simulink model "SecRwLtStLgrstUpwdDnwdCtrl"  (R2018b)
settings: Solver=FixedStepDiscrete  StartTime=0.0  StopTime=10.0  FixedStep=0.01  RelTol=1e-3
undefined symbols (not defined in the file or in its folder): KeSMSuMdMotFinshdTm_Val, KeSMSuMdRetryTm1_Val, KeSMSuModeReqDurgTm_Val, KeSMSwSecRwLtStLgrstUpwdDnwdEnTrigBitMask_Val
libraries: StCtrlLibBkRecln x1
settings Model: Creator=sn2xws  LastModifiedBy=sn55gm
settings Model: ModifiedHistory=|
  | 2024.10.14 V3.0.0 bitmask接口改为变量接口
  | 25.7.7 V3.13.0 Md61 Md62新增Retry口
settings DataIOCC: SaveFormat=StructureWithTime
settings OptimizationCC: DefaultParameterBehavior=Inlined  EnhancedBackFolding=on  PassReuseOutputArgsAs=Individual arguments  ZeroExternalMemoryAtStartup=off  ZeroInternalMemoryAtStartup=off  OptimizeBlockOrder=speed  DifferentSizesBufferReuse=on  OptimizationCustomize=off
settings DebuggingCC: ParameterTunabilityLossMsg=error
settings ModelReferenceCC: ModelReferenceNumInstancesAllowed=Single
settings SFSimCC: MATLABDynamicMemAlloc=off
settings RTWCC: SystemTargetFile=autosar.tlc  GenCodeOnly=on  TemplateMakefile=ert_default_tmf  Description=AUTOSAR  GenerateReport=on  IncludeHyperlinkInReport=on  LaunchReport=on  GenerateTraceInfo=on  GenerateTraceReport=on  GenerateTraceReportSl=on  GenerateTraceReportSf=on  GenerateTraceReportEml=on
settings CodeAppCC: ForceParamTrailComments=on  IgnoreCustomStorageClasses=off  OperatorAnnotations=on  SimulinkDataObjDesc=on  SFDataObjDesc=on  InsertBlockDesc=on
settings STFCustomTargetCC: TargetLangStandard=C99 (ISO)  MultiwordLength=256  ParMdlRefBuildCompliant=on  CompOptLevelCompliant=on  IncludeMdlTerminateFcn=off  CombineOutputUpdateFcns=on  SuppressErrorStatus=on  ERTCustomFileBanners=on  SupportNonFinite=off  SupportComplex=off  SupportContinuousTime=off  SupportNonInlinedSFcns=off  RemoveResetFunc=on  MATLABClassNameForMDSCustomization=Simulink.SoftwareTarget.ERTCustomization  AutosarCompliant=on  UseToolchainInfoCompliant=on  LookupTableObjectStructAxisOrder=2,1,3,4,...  LUTObjectStructOrderEvenSpacing=Size,Table,Breakpoints  SystemTargetFile=autosar.tlc
settings ERTTargetCC: TargetLangStandard=C99 (ISO)  ConcurrentExecutionCompliant=off  IncludeMdlTerminateFcn=off  SuppressErrorStatus=on  SupportNonFinite=off  SupportComplex=off  ModelStepFunctionPrototypeControlCompliant=off  CPPClassGenCompliant=off  AutosarCompliant=on  LookupTableObjectStructAxisOrder=2,1,3,4,...  LUTObjectStructOrderEvenSpacing=Size,Table,Breakpoints  InlinedParameterPlacement=NonHierarchical  ERTCustomFileTemplate=example_file_process.tlc  ERTFilePackagingFormat=Compact

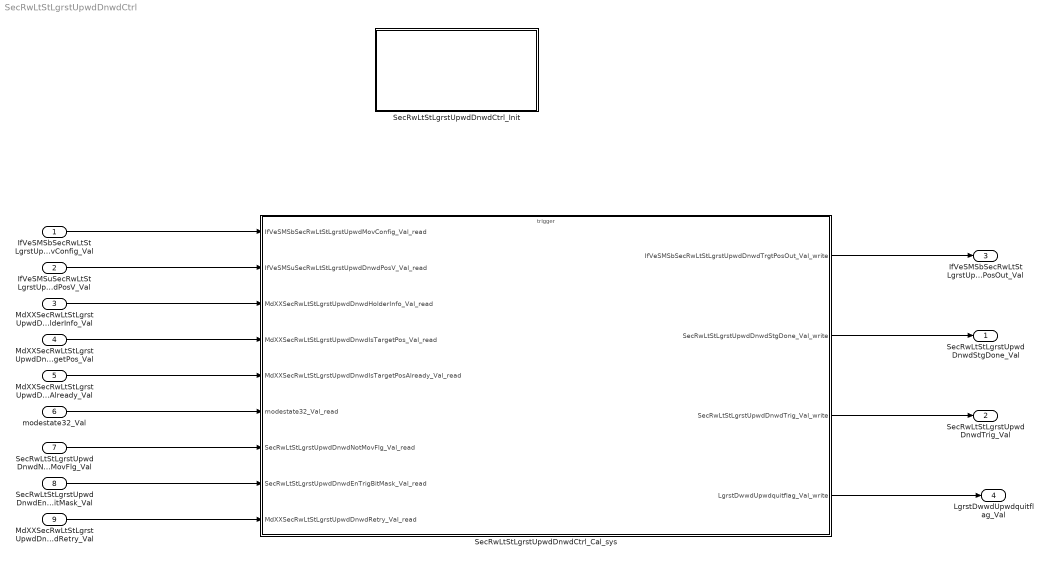
== system SecRwLtStLgrstUpwdDnwdCtrl ==
  IfVeSMSbSecRwLtStLgrstUpwdMovConfig_Val : Inport  OutDataTypeStr=boolean  PortDimensions=1
  IfVeSMSuSecRwLtStLgrstUpwdDnwdPosV_Val : Inport  Port=2  OutDataTypeStr=boolean  PortDimensions=1
  MdXXSecRwLtStLgrstUpwdDnwdHolderInfo_Val : Inport  Port=3  OutDataTypeStr=uint32  PortDimensions=1
  MdXXSecRwLtStLgrstUpwdDnwdIsTargetPos_Val : Inport  Port=4  OutDataTypeStr=uint32  PortDimensions=1
  MdXXSecRwLtStLgrstUpwdDnwdIsTargetPosAlready_Val : Inport  Port=5  OutDataTypeStr=uint32  PortDimensions=1
  modestate32_Val : Inport  Port=6  OutDataTypeStr=uint32  PortDimensions=1
  SecRwLtStLgrstUpwdDnwdNotMovFlg_Val : Inport  Port=7  OutDataTypeStr=boolean  PortDimensions=1
  SecRwLtStLgrstUpwdDnwdEnTrigBitMask_Val : Inport  Port=8  OutDataTypeStr=uint32  PortDimensions=1
  MdXXSecRwLtStLgrstUpwdDnwdRetry_Val : Inport  Port=9  OutDataTypeStr=uint32  PortDimensions=1
  SecRwLtStLgrstUpwdDnwdCtrl_Cal_sys : Subsystem
  SecRwLtStLgrstUpwdDnwdCtrl_Init : Subsystem
  SecRwLtStLgrstUpwdDnwdStgDone_Val : Outport  OutDataTypeStr=boolean  PortDimensions=1
  SecRwLtStLgrstUpwdDnwdTrig_Val : Outport  Port=2  OutDataTypeStr=boolean  PortDimensions=1
  IfVeSMSbSecRwLtStLgrstUpwdDnwdTrgtPosOut_Val : Outport  Port=3  OutDataTypeStr=boolean  PortDimensions=1
  LgrstDwwdUpwdquitflag_Val : Outport  Port=4  OutDataTypeStr=boolean  PortDimensions=1
  wires:
  IfVeSMSbSecRwLtStLgrstUpwdMovConfig_Val/1 -> SecRwLtStLgrstUpwdDnwdCtrl_Cal_sys/1(IfVeSMSbSecRwLtStLgrstUpwdMovConfig_Val_read)
  IfVeSMSuSecRwLtStLgrstUpwdDnwdPosV_Val/1 -> SecRwLtStLgrstUpwdDnwdCtrl_Cal_sys/2(IfVeSMSuSecRwLtStLgrstUpwdDnwdPosV_Val_read)
  MdXXSecRwLtStLgrstUpwdDnwdHolderInfo_Val/1 -> SecRwLtStLgrstUpwdDnwdCtrl_Cal_sys/3(MdXXSecRwLtStLgrstUpwdDnwdHolderInfo_Val_read)
  MdXXSecRwLtStLgrstUpwdDnwdIsTargetPos_Val/1 -> SecRwLtStLgrstUpwdDnwdCtrl_Cal_sys/4(MdXXSecRwLtStLgrstUpwdDnwdIsTargetPos_Val_read)
  MdXXSecRwLtStLgrstUpwdDnwdIsTargetPosAlready_Val/1 -> SecRwLtStLgrstUpwdDnwdCtrl_Cal_sys/5(MdXXSecRwLtStLgrstUpwdDnwdIsTargetPosAlready_Val_read)
  modestate32_Val/1 -> SecRwLtStLgrstUpwdDnwdCtrl_Cal_sys/6(modestate32_Val_read)
  SecRwLtStLgrstUpwdDnwdNotMovFlg_Val/1 -> SecRwLtStLgrstUpwdDnwdCtrl_Cal_sys/7(SecRwLtStLgrstUpwdDnwdNotMovFlg_Val_read)
  SecRwLtStLgrstUpwdDnwdCtrl_Cal_sys/1(IfVeSMSbSecRwLtStLgrstUpwdDnwdTrgtPosOut_Val_write) -> IfVeSMSbSecRwLtStLgrstUpwdDnwdTrgtPosOut_Val/1
  SecRwLtStLgrstUpwdDnwdCtrl_Cal_sys/2(SecRwLtStLgrstUpwdDnwdStgDone_Val_write) -> SecRwLtStLgrstUpwdDnwdStgDone_Val/1
  SecRwLtStLgrstUpwdDnwdCtrl_Cal_sys/3(SecRwLtStLgrstUpwdDnwdTrig_Val_write) -> SecRwLtStLgrstUpwdDnwdTrig_Val/1
  SecRwLtStLgrstUpwdDnwdEnTrigBitMask_Val/1 -> SecRwLtStLgrstUpwdDnwdCtrl_Cal_sys/8(SecRwLtStLgrstUpwdDnwdEnTrigBitMask_Val_read)
  MdXXSecRwLtStLgrstUpwdDnwdRetry_Val/1 -> SecRwLtStLgrstUpwdDnwdCtrl_Cal_sys/9(MdXXSecRwLtStLgrstUpwdDnwdRetry_Val_read)
  SecRwLtStLgrstUpwdDnwdCtrl_Cal_sys/4(LgrstDwwdUpwdquitflag_Val_write) -> LgrstDwwdUpwdquitflag_Val/1

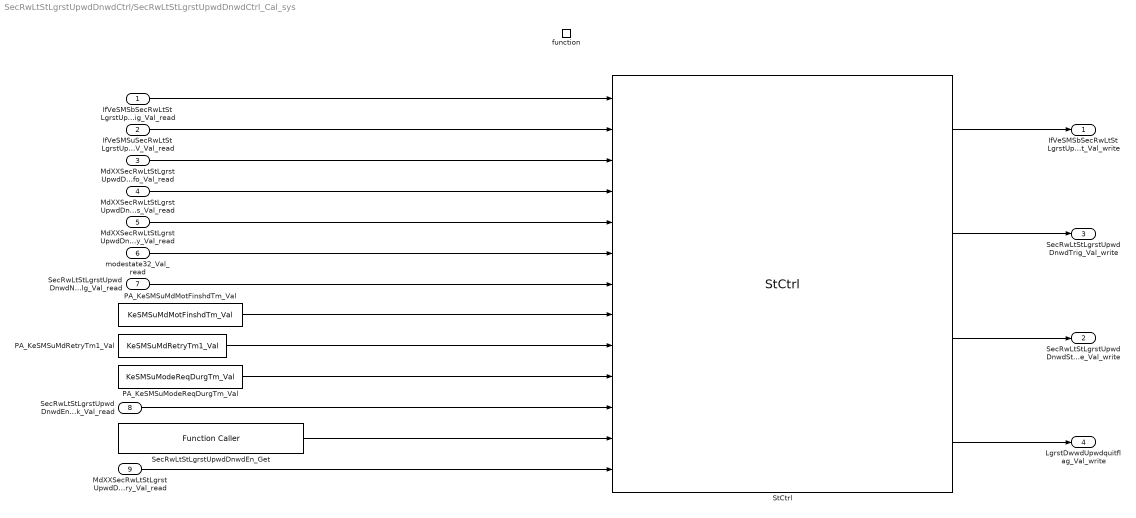
== system SecRwLtStLgrstUpwdDnwdCtrl/SecRwLtStLgrstUpwdDnwdCtrl_Cal_sys ==
  IfVeSMSbSecRwLtStLgrstUpwdMovConfig_Val_read : Inport
  IfVeSMSuSecRwLtStLgrstUpwdDnwdPosV_Val_read : Inport  Port=2
  MdXXSecRwLtStLgrstUpwdDnwdHolderInfo_Val_read : Inport  Port=3
  MdXXSecRwLtStLgrstUpwdDnwdIsTargetPos_Val_read : Inport  Port=4
  MdXXSecRwLtStLgrstUpwdDnwdIsTargetPosAlready_Val_read : Inport  Port=5
  modestate32_Val_read : Inport  Port=6
  SecRwLtStLgrstUpwdDnwdNotMovFlg_Val_read : Inport  Port=7
  SecRwLtStLgrstUpwdDnwdEnTrigBitMask_Val_read : Inport  Port=8
  MdXXSecRwLtStLgrstUpwdDnwdRetry_Val_read : Inport  Port=9
  function : TriggerPort  TriggerType=function-call  IsSimulinkFunction=on  FunctionName=SecRwLtStLgrstUpwdDnwdCtrl_Cal  VariantControl=(inherit)
  PA_KeSMSuMdMotFinshdTm_Val : Constant  Value=KeSMSuMdMotFinshdTm_Val
  PA_KeSMSuMdRetryTm1_Val : Constant  Value=KeSMSuMdRetryTm1_Val
  PA_KeSMSuModeReqDurgTm_Val : Constant  Value=KeSMSuModeReqDurgTm_Val
  SecRwLtStLgrstUpwdDnwdEn_Get : FunctionCaller  FunctionPrototype=data = SecRwLtStLgrstUpwdDnwdEn_Get()  OutputArgumentSpecifications=uint32(1)
  StCtrl : StCtrlLibBkRecln/StCtrl  SystemSampleTime=-1
  IfVeSMSbSecRwLtStLgrstUpwdDnwdTrgtPosOut_Val_write : Outport
      settings: EnsureOutportIsVirtual=on
  SecRwLtStLgrstUpwdDnwdStgDone_Val_write : Outport  Port=2
      settings: EnsureOutportIsVirtual=on
  SecRwLtStLgrstUpwdDnwdTrig_Val_write : Outport  Port=3
      settings: EnsureOutportIsVirtual=on
  LgrstDwwdUpwdquitflag_Val_write : Outport  Port=4
      settings: EnsureOutportIsVirtual=on
  wires:
  StCtrl/1 -> IfVeSMSbSecRwLtStLgrstUpwdDnwdTrgtPosOut_Val_write/1
  StCtrl/2 -> SecRwLtStLgrstUpwdDnwdTrig_Val_write/1
  StCtrl/3 -> SecRwLtStLgrstUpwdDnwdStgDone_Val_write/1
  IfVeSMSbSecRwLtStLgrstUpwdMovConfig_Val_read/1 -> StCtrl/1
  IfVeSMSuSecRwLtStLgrstUpwdDnwdPosV_Val_read/1 -> StCtrl/2
  MdXXSecRwLtStLgrstUpwdDnwdHolderInfo_Val_read/1 -> StCtrl/3
  MdXXSecRwLtStLgrstUpwdDnwdIsTargetPos_Val_read/1 -> StCtrl/4
  MdXXSecRwLtStLgrstUpwdDnwdIsTargetPosAlready_Val_read/1 -> StCtrl/5
  modestate32_Val_read/1 -> StCtrl/6
  SecRwLtStLgrstUpwdDnwdNotMovFlg_Val_read/1 -> StCtrl/7
  SecRwLtStLgrstUpwdDnwdEnTrigBitMask_Val_read/1 -> StCtrl/11
  SecRwLtStLgrstUpwdDnwdEn_Get/1 -> StCtrl/12
  PA_KeSMSuMdMotFinshdTm_Val/1 -> StCtrl/8
  PA_KeSMSuModeReqDurgTm_Val/1 -> StCtrl/10
  PA_KeSMSuMdRetryTm1_Val/1 -> StCtrl/9
  MdXXSecRwLtStLgrstUpwdDnwdRetry_Val_read/1 -> StCtrl/13
  StCtrl/4 -> LgrstDwwdUpwdquitflag_Val_write/1

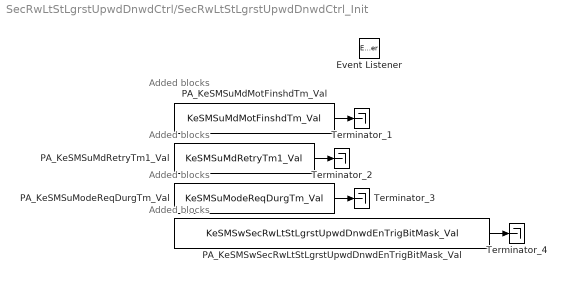
== system SecRwLtStLgrstUpwdDnwdCtrl/SecRwLtStLgrstUpwdDnwdCtrl_Init ==
  note: Added blocks
  note: Added blocks
  note: Added blocks
  note: Added blocks
  Event Listener : EventListener  EventName=reset
  PA_KeSMSuMdMotFinshdTm_Val : Constant  Value=KeSMSuMdMotFinshdTm_Val
  PA_KeSMSuMdRetryTm1_Val : Constant  Value=KeSMSuMdRetryTm1_Val
  PA_KeSMSuModeReqDurgTm_Val : Constant  Value=KeSMSuModeReqDurgTm_Val
  PA_KeSMSwSecRwLtStLgrstUpwdDnwdEnTrigBitMask_Val : Constant  Value=KeSMSwSecRwLtStLgrstUpwdDnwdEnTrigBitMask_Val
  Terminator_{1..4} (4 alike) : Terminator
  wires:
  PA_KeSMSuMdMotFinshdTm_Val/1 -> Terminator_1/1
  PA_KeSMSuMdRetryTm1_Val/1 -> Terminator_2/1
  PA_KeSMSuModeReqDurgTm_Val/1 -> Terminator_3/1
  PA_KeSMSwSecRwLtStLgrstUpwdDnwdEnTrigBitMask_Val/1 -> Terminator_4/1
